simulink library "helperLib"  (R2014b)
settings: Solver=ode45  StartTime=0.0  StopTime=10.0  RelTol=1e-3
values from neighbouring files (symbols this model uses):
  atanDomain = 6    [rev0BB_setup.m]
  atanResolution = 2^-7    (= 0.0078125)    [rev0BB_setup.m]
  averaging_denom = zeros(1, averaging_samples)    [rev0BB_setup.m]
  averaging_num = (1/averaging_samples).*ones(1, averaging_samples)    [rev0BB_setup.m]
libraries: helperLib x11, simulink x8, dspsigops x7
settings Model: Creator=cyarp  LastModifiedBy=cyarp

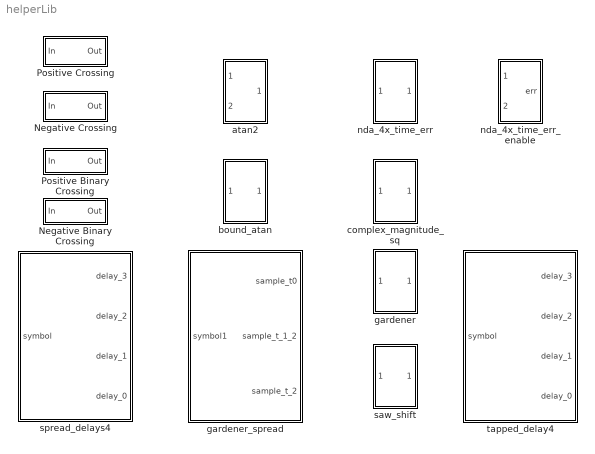
== system helperLib ==
  Negative Binary Crossing : Subsystem
  Negative Crossing : Subsystem  mask{crossPt=0}
      mask prompts: crossPt "Crossing Point"
      mask help:
      | Negative Crossing
      | Will output true if goes greater than or equal to threshold to less than
      | theshold.  Will output zero otherwise.
      mask Display: fprintf('-Cross (%d)', crossPt)
  Positive Binary Crossing : Subsystem
  Positive Crossing : Subsystem  mask{crossPt=0}
      mask prompts: crossPt "Crossing Pt"
      mask help:
      | Positive Crossing
      | Will output true if goes from below threshold to greater than or equal to
      | theshold.  Will output zero otherwise.
      mask Display: fprintf('+Cross (%d)', crossPt)
  atan2 : Subsystem
  bound_atan : Subsystem
  complex_magnitude_sq : Subsystem
  gardener : Subsystem
  gardener_spread : Subsystem
  nda_4x_time_err : Subsystem
  nda_4x_time_err_enable : Subsystem
  saw_shift : Subsystem
  spread_delays4 : Subsystem
  "tapped_delay4 " : Subsystem

== system helperLib/Negative Binary Crossing ==
  In : Inport  OutDataTypeStr=boolean
  Delay : Delay  DelayLength=1  InitialCondition=0
  Logical Operator : Logic  AllPortsSameDT=off  OutDataTypeStr=boolean
  Logical Operator1 : Logic  Operator=NOT  Inputs=1  AllPortsSameDT=off  OutDataTypeStr=boolean
  Out : Outport  OutDataTypeStr=boolean
  wires:
  In/1 -> Logical Operator1/1, Delay/1
  Logical Operator/1 -> Out/1
  Logical Operator1/1 -> Logical Operator/1
  Delay/1 -> Logical Operator/2

== system helperLib/Negative Crossing ==
  In : Inport
  Compare To Constant : simulink/Logic and Bit Operations/Compare To Constant  relop=<  const=crossPt  OutDataTypeStr=boolean
  Compare To Constant1 : simulink/Logic and Bit Operations/Compare To Constant  relop=>=  const=crossPt  OutDataTypeStr=boolean
  Delay : Delay  DelayLength=1  InitialCondition=0
  Logical Operator : Logic  AllPortsSameDT=off  OutDataTypeStr=boolean
  Out : Outport  OutDataTypeStr=boolean
  wires:
  Logical Operator/1 -> Out/1
  In/1 -> Compare To Constant1/1, Compare To Constant/1
  Compare To Constant/1 -> Logical Operator/1
  Compare To Constant1/1 -> Delay/1
  Delay/1 -> Logical Operator/2

== system helperLib/Positive Binary Crossing ==
  In : Inport  OutDataTypeStr=boolean
  Delay : Delay  DelayLength=1  InitialCondition=0
  Logical Operator : Logic  AllPortsSameDT=off  OutDataTypeStr=boolean
  Logical Operator1 : Logic  Operator=NOT  Inputs=1  AllPortsSameDT=off  OutDataTypeStr=boolean
  Out : Outport  OutDataTypeStr=boolean
  wires:
  In/1 -> Logical Operator/1, Delay/1
  Logical Operator/1 -> Out/1
  Delay/1 -> Logical Operator1/1
  Logical Operator1/1 -> Logical Operator/2

== system helperLib/Positive Crossing ==
  In : Inport
  Compare To Constant : simulink/Logic and Bit Operations/Compare To Constant  relop=>=  const=crossPt  OutDataTypeStr=boolean
  Compare To Constant1 : simulink/Logic and Bit Operations/Compare To Constant  relop=<  const=crossPt  OutDataTypeStr=boolean
  Delay : Delay  DelayLength=1  InitialCondition=0
  Logical Operator : Logic  AllPortsSameDT=off  OutDataTypeStr=boolean
  Out : Outport  OutDataTypeStr=boolean
  wires:
  Compare To Constant1/1 -> Delay/1
  Compare To Constant/1 -> Logical Operator/1
  Logical Operator/1 -> Out/1
  In/1 -> Compare To Constant1/1, Compare To Constant/1
  Delay/1 -> Logical Operator/2

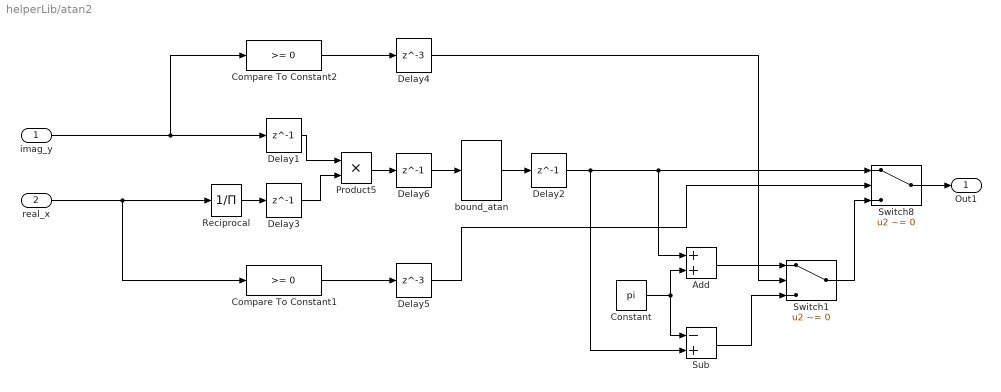
== system helperLib/atan2 ==
  imag_y : Inport
  real_x : Inport  Port=2
  Add : Sum
  Compare To Constant1 : simulink/Logic and Bit Operations/Compare To Constant  relop=>=  const=0  OutDataTypeStr=boolean
  Compare To Constant2 : simulink/Logic and Bit Operations/Compare To Constant  relop=>=  const=0  OutDataTypeStr=boolean
  Constant : Constant  Value=pi  OutDataTypeStr=Inherit: Inherit via back propagation
  Delay{1..3,6} (4 alike) : Delay  DelayLength=1  InitialCondition=0
  Delay4 : Delay  DelayLength=3  InitialCondition=0
  Delay5 : Delay  DelayLength=3  InitialCondition=0
  Product5 : Product  OutDataTypeStr=Inherit: Same as first input
  Reciprocal : Product  Inputs=/  SaturateOnIntegerOverflow=on  RndMeth=Zero
  Sub : Sum  Inputs=-+
  Switch1 : Switch  Criteria=u2 ~= 0  OutDataTypeStr=Inherit: Inherit via back propagation
  Switch8 : Switch  Criteria=u2 ~= 0  OutDataTypeStr=Inherit: Inherit via back propagation
  bound_atan : helperLib/bound_atan
  Out1 : Outport
  wires:
  Product5/1 -> Delay6/1
  Delay3/1 -> Product5/2
  Delay6/1 -> bound_atan/1
  Reciprocal/1 -> Delay3/1
  bound_atan/1 -> Delay2/1
  Delay1/1 -> Product5/1
  Delay2/1 -> Sub/2, Add/1, Switch8/1
  Compare To Constant1/1 -> Delay5/1
  Compare To Constant2/1 -> Delay4/1
  Switch1/1 -> Switch8/3
  Add/1 -> Switch1/1
  Constant/1 -> Add/2, Sub/1
  Sub/1 -> Switch1/3
  Switch8/1 -> Out1/1
  imag_y/1 -> Compare To Constant2/1, Delay1/1
  real_x/1 -> Compare To Constant1/1, Reciprocal/1
  Delay5/1 -> Switch8/2
  Delay4/1 -> Switch1/2

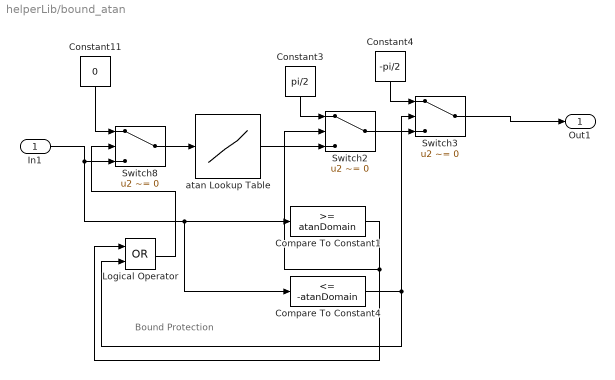
== system helperLib/bound_atan ==
  note: Bound Protection
  In1 : Inport
  Compare To Constant1 : simulink/Logic and Bit Operations/Compare To Constant  relop=>=  const=atanDomain  OutDataTypeStr=boolean
  Compare To Constant4 : simulink/Logic and Bit Operations/Compare To Constant  relop=<=  const=-atanDomain  OutDataTypeStr=boolean
  Constant11 : Constant  Value=0  OutDataTypeStr=Inherit: Inherit via back propagation
  Constant3 : Constant  Value=pi/2  OutDataTypeStr=Inherit: Inherit via back propagation
  Constant4 : Constant  Value=-pi/2  OutDataTypeStr=Inherit: Inherit via back propagation
  Logical Operator : Logic  Operator=OR  AllPortsSameDT=off  OutDataTypeStr=boolean
  Switch2 : Switch  Criteria=u2 ~= 0  OutDataTypeStr=Inherit: Inherit via back propagation
  Switch3 : Switch  Criteria=u2 ~= 0  OutDataTypeStr=Inherit: Inherit via back propagation
  Switch8 : Switch  Criteria=u2 ~= 0  OutDataTypeStr=Inherit: Inherit via back propagation
  atan Lookup Table : Lookup_n-D  NumberOfTableDimensions=1  BreakpointsForDimension1=[-atanDomain:atanResolution:atanDomain]  IndexSearchMethod=Evenly spaced points  Table=atan([-atanDomain:atanResolution:atanDomain])  InterpMethod=Flat  DiagnosticForOutOfRangeInput=Error  InternalRulePriority=Speed  OutDataTypeStr=fixdt(1,30,26)  RndMeth=Simplest  InputSameDT=on
  Out1 : Outport
  wires:
  Compare To Constant1/1 -> Switch2/2, Logical Operator/1
  Compare To Constant4/1 -> Logical Operator/2, Switch3/2
  atan Lookup Table/1 -> Switch2/3
  Constant3/1 -> Switch2/1
  Switch2/1 -> Switch3/3
  Constant4/1 -> Switch3/1
  Switch3/1 -> Out1/1
  In1/1 -> Switch8/3, Compare To Constant1/1, Compare To Constant4/1
  Logical Operator/1 -> Switch8/2
  Constant11/1 -> Switch8/1
  Switch8/1 -> atan Lookup Table/1

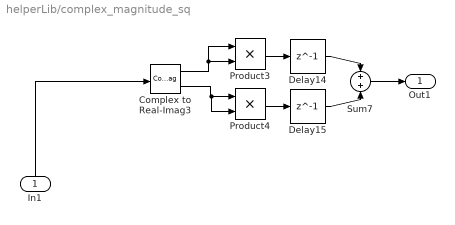
== system helperLib/complex_magnitude_sq ==
  In1 : Inport
  Complex to Real-Imag3 : ComplexToRealImag
  Delay14 : Delay  DelayLength=1  InitialCondition=0
  Delay15 : Delay  DelayLength=1  InitialCondition=0
  Product3 : Product
  Product4 : Product
  Sum7 : Sum  OutDataTypeStr=Inherit: Same as first input
  Out1 : Outport
  wires:
  Product3/1 -> Delay14/1
  Product4/1 -> Delay15/1
  Sum7/1 -> Out1/1
  Delay15/1 -> Sum7/2
  Delay14/1 -> Sum7/1
  In1/1 -> Complex to Real-Imag3/1
  Complex to Real-Imag3/1 -> Product3/2, Product3/1
  Complex to Real-Imag3/2 -> Product4/2, Product4/1

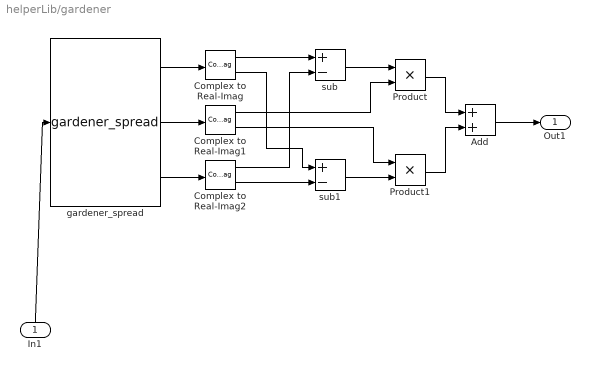
== system helperLib/gardener ==
  In1 : Inport
  Add : Sum
  Complex to Real-Imag : ComplexToRealImag
  Complex to Real-Imag1 : ComplexToRealImag
  Complex to Real-Imag2 : ComplexToRealImag
  Product : Product
  Product1 : Product
  gardener_spread : helperLib/gardener_spread
  sub : Sum  Inputs=+-
  sub1 : Sum  Inputs=+-
  Out1 : Outport
  wires:
  gardener_spread/2 -> Complex to Real-Imag1/1
  gardener_spread/1 -> Complex to Real-Imag/1
  Complex to Real-Imag2/2 -> sub1/2
  gardener_spread/3 -> Complex to Real-Imag2/1
  Complex to Real-Imag2/1 -> sub/2
  Complex to Real-Imag1/2 -> Product1/1
  Add/1 -> Out1/1
  sub1/1 -> Product1/2
  Complex to Real-Imag1/1 -> Product/2
  Complex to Real-Imag/1 -> sub/1
  Product/1 -> Add/1
  Complex to Real-Imag/2 -> sub1/1
  sub/1 -> Product/1
  Product1/1 -> Add/2
  In1/1 -> gardener_spread/1

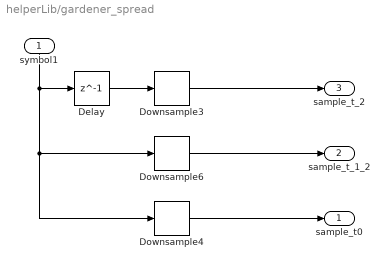
== system helperLib/gardener_spread ==
  symbol1 : Inport
  Delay : Delay  DelayLength=1  InitialCondition=0
  Downsample3 : dspsigops/Downsample  N=4  phase=0  InputProcessing=Columns as channels (frame based)  RateOptions=Allow multirate processing  smode=Allow multirate  fmode=Maintain input frame size  ic=0
  Downsample4 : dspsigops/Downsample  N=4  phase=0  InputProcessing=Columns as channels (frame based)  RateOptions=Allow multirate processing  smode=Allow multirate  fmode=Maintain input frame size  ic=0
  Downsample6 : dspsigops/Downsample  N=4  phase=2  InputProcessing=Columns as channels (frame based)  RateOptions=Allow multirate processing  smode=Allow multirate  fmode=Maintain input frame size  ic=0
  sample_t0 : Outport
  sample_t_1_2 : Outport  Port=2
  sample_t_2 : Outport  Port=3
  wires:
  symbol1/1 -> Delay/1, Downsample4/1, Downsample6/1
  Downsample6/1 -> sample_t_1_2/1
  Downsample4/1 -> sample_t0/1
  Downsample3/1 -> sample_t_2/1
  Delay/1 -> Downsample3/1

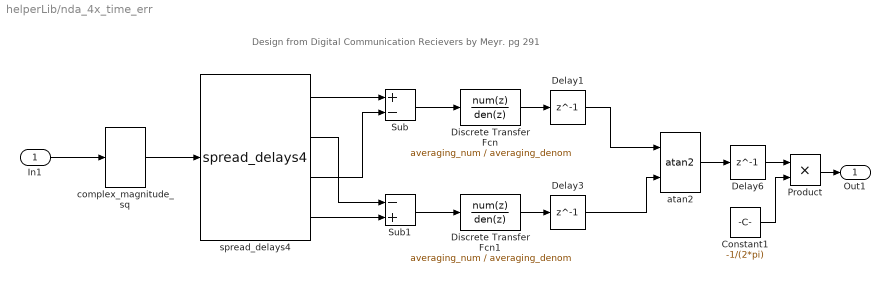
== system helperLib/nda_4x_time_err ==
  note: Design from Digital Communication Recievers by Meyr. pg 291
  In1 : Inport
  Constant1 : Constant  Value=-1/(2*pi)  OutDataTypeStr=Inherit: Inherit via back propagation
  Delay1 : Delay  DelayLength=1  InitialCondition=0
  Delay3 : Delay  DelayLength=1  InitialCondition=0
  Delay6 : Delay  DelayLength=1  InitialCondition=0
  Discrete Transfer Fcn : DiscreteTransferFcn  Numerator=averaging_num  Denominator=averaging_denom  OutDataTypeStr=Inherit: Same as input
  Discrete Transfer Fcn1 : DiscreteTransferFcn  Numerator=averaging_num  Denominator=averaging_denom  OutDataTypeStr=Inherit: Same as input
  Product : Product
  Sub : Sum  Inputs=+-
  Sub1 : Sum  Inputs=-+
  atan2 : helperLib/atan2
  complex_magnitude_sq : helperLib/complex_magnitude_sq
  spread_delays4 : helperLib/spread_delays4
  Out1 : Outport
  wires:
  atan2/1 -> Delay6/1
  Sub1/1 -> Discrete Transfer Fcn1/1
  Constant1/1 -> Product/2
  spread_delays4/4 -> Sub1/2
  spread_delays4/1 -> Sub/1
  Delay6/1 -> Product/1
  Sub/1 -> Discrete Transfer Fcn/1
  complex_magnitude_sq/1 -> spread_delays4/1
  spread_delays4/2 -> Sub1/1
  Discrete Transfer Fcn/1 -> Delay1/1
  Delay1/1 -> atan2/1
  Product/1 -> Out1/1
  spread_delays4/3 -> Sub/2
  In1/1 -> complex_magnitude_sq/1
  Discrete Transfer Fcn1/1 -> Delay3/1
  Delay3/1 -> atan2/2

== system helperLib/nda_4x_time_err_enable ==
  note: Design from Digital Communication Recievers by Meyr. pg 291, 529
  samples : Inport
  enable : Inport  Port=2
  phase_est : Subsystem
  "tapped_delay4 " : helperLib/tapped_delay4 
  err : Outport
  wires:
  samples/1 -> "tapped_delay4 "/1
  enable/1 -> phase_est/Enable
  "tapped_delay4 "/1 -> phase_est/1(In1)
  "tapped_delay4 "/2 -> phase_est/2(In2)
  "tapped_delay4 "/3 -> phase_est/3(In3)
  "tapped_delay4 "/4 -> phase_est/4(In4)
  phase_est/1(Out1) -> err/1

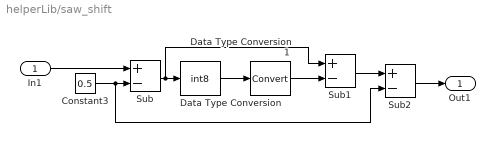
== system helperLib/saw_shift ==
  In1 : Inport
  Constant3 : Constant  Value=0.5  OutDataTypeStr=Inherit: Inherit via back propagation
  Data Type Conversion : DataTypeConversion  OutDataTypeStr=int8
  Data Type Conversion1 : DataTypeConversion
  Sub : Sum  Inputs=+-
  Sub1 : Sum  Inputs=+-
  Sub2 : Sum  Inputs=+-
  Out1 : Outport
  wires:
  Sub1/1 -> Sub2/1
  Constant3/1 -> Sub2/2, Sub/2
  Sub/1 -> Sub1/1, Data Type Conversion/1
  Data Type Conversion1/1 -> Sub1/2
  In1/1 -> Sub/1
  Data Type Conversion/1 -> Data Type Conversion1/1
  Sub2/1 -> Out1/1

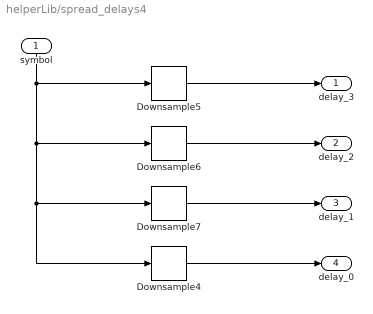
== system helperLib/spread_delays4 ==
  symbol : Inport
  Downsample4 : dspsigops/Downsample  N=4  phase=0  InputProcessing=Columns as channels (frame based)  RateOptions=Allow multirate processing  smode=Allow multirate  fmode=Maintain input frame size  ic=0
  Downsample5 : dspsigops/Downsample  N=4  phase=3  InputProcessing=Columns as channels (frame based)  RateOptions=Allow multirate processing  smode=Allow multirate  fmode=Maintain input frame size  ic=0
  Downsample6 : dspsigops/Downsample  N=4  phase=2  InputProcessing=Columns as channels (frame based)  RateOptions=Allow multirate processing  smode=Allow multirate  fmode=Maintain input frame size  ic=0
  Downsample7 : dspsigops/Downsample  N=4  phase=1  InputProcessing=Columns as channels (frame based)  RateOptions=Allow multirate processing  smode=Allow multirate  fmode=Maintain input frame size  ic=0
  delay_3 : Outport
  delay_2 : Outport  Port=2
  delay_1 : Outport  Port=3
  delay_0 : Outport  Port=4
  wires:
  symbol/1 -> Downsample4/1, Downsample7/1, Downsample6/1, Downsample5/1
  Downsample5/1 -> delay_3/1
  Downsample6/1 -> delay_2/1
  Downsample7/1 -> delay_1/1
  Downsample4/1 -> delay_0/1

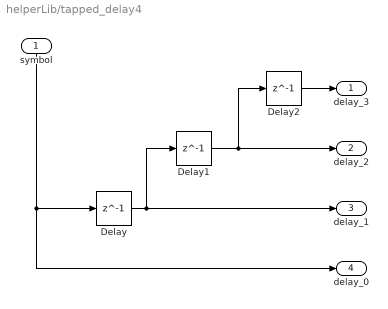
== system helperLib/tapped_delay4  ==
  symbol : Inport
  Delay : Delay  DelayLength=1  InitialCondition=0
  Delay1 : Delay  DelayLength=1  InitialCondition=0
  Delay2 : Delay  DelayLength=1  InitialCondition=0
  delay_3 : Outport
  delay_2 : Outport  Port=2
  delay_1 : Outport  Port=3
  delay_0 : Outport  Port=4
  wires:
  symbol/1 -> Delay/1, delay_0/1
  Delay/1 -> Delay1/1, delay_1/1
  Delay1/1 -> Delay2/1, delay_2/1
  Delay2/1 -> delay_3/1

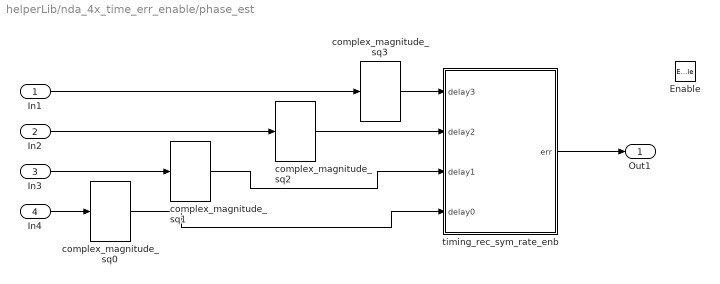
== system helperLib/nda_4x_time_err_enable/phase_est ==
  In1 : Inport
  In2 : Inport  Port=2
  In3 : Inport  Port=3
  In4 : Inport  Port=4
  Enable : EnablePort
  complex_magnitude_sq{0..3} (4 alike) : helperLib/complex_magnitude_sq
  timing_rec_sym_rate_enb : Subsystem
  Out1 : Outport
  wires:
  In1/1 -> complex_magnitude_sq3/1
  In2/1 -> complex_magnitude_sq2/1
  timing_rec_sym_rate_enb/1(err) -> Out1/1
  complex_magnitude_sq3/1 -> timing_rec_sym_rate_enb/1(delay3)
  complex_magnitude_sq2/1 -> timing_rec_sym_rate_enb/2(delay2)
  complex_magnitude_sq0/1 -> timing_rec_sym_rate_enb/4(delay0)
  complex_magnitude_sq1/1 -> timing_rec_sym_rate_enb/3(delay1)
  In3/1 -> complex_magnitude_sq1/1
  In4/1 -> complex_magnitude_sq0/1

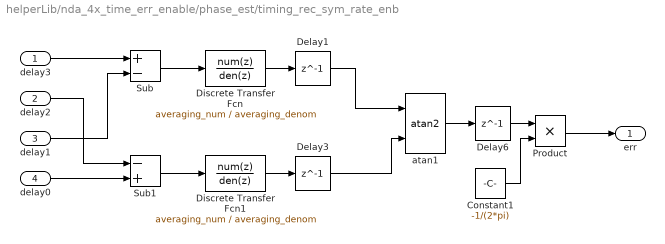
== system helperLib/nda_4x_time_err_enable/phase_est/timing_rec_sym_rate_enb ==
  delay3 : Inport
  delay2 : Inport  Port=2
  delay1 : Inport  Port=3
  delay0 : Inport  Port=4
  Constant1 : Constant  Value=-1/(2*pi)  OutDataTypeStr=Inherit: Inherit via back propagation
  Delay1 : Delay  DelayLength=1  InitialCondition=0
  Delay3 : Delay  DelayLength=1  InitialCondition=0
  Delay6 : Delay  DelayLength=1  InitialCondition=0
  Discrete Transfer Fcn : DiscreteTransferFcn  Numerator=averaging_num  Denominator=averaging_denom  OutDataTypeStr=Inherit: Same as input
  Discrete Transfer Fcn1 : DiscreteTransferFcn  Numerator=averaging_num  Denominator=averaging_denom  OutDataTypeStr=Inherit: Same as input
  Product : Product
  Sub : Sum  Inputs=+-
  Sub1 : Sum  Inputs=-+
  atan1 : helperLib/atan2
  err : Outport
  wires:
  Delay3/1 -> atan1/2
  Sub/1 -> Discrete Transfer Fcn/1
  Discrete Transfer Fcn/1 -> Delay1/1
  delay2/1 -> Sub1/1
  Product/1 -> err/1
  Delay1/1 -> atan1/1
  delay1/1 -> Sub/2
  Discrete Transfer Fcn1/1 -> Delay3/1
  atan1/1 -> Delay6/1
  Sub1/1 -> Discrete Transfer Fcn1/1
  Constant1/1 -> Product/2
  delay0/1 -> Sub1/2
  delay3/1 -> Sub/1
  Delay6/1 -> Product/1
